simulink model "dspaudiosrc_fixpt"  (Simulink 8.3)
settings: Solver=FixedStepDiscrete  SolverMode=SingleTasking  StartTime=0.0  StopTime=inf  RelTol=1e-3
model workspace (MATLAB code in the model file):
  | load dspaudiosrc
libraries: dspmlti4 x1, dspsigops x1, dspsrcs4 x1, dspmisc x1
settings Model: Creator=The MathWorks Inc.  ExtModeAutoUpdateStatusClock=off
settings DataIOCC: SaveOutput=off  SignalLogging=off  SaveTime=off
settings OptimizationCC: InlineParams=on  ExpressionDepthLimit=2147483647  InitFltsAndDblsToZero=on
settings DebuggingCC: SignalResolutionControl=TryResolveAllWithWarning  SolverPrmCheckMsg=none  MultiTaskDSMMsg=warning  MultiTaskCondExecSysMsg=none  IntegerOverflowMsg=none  ParameterPrecisionLossMsg=none  FcnCallInpInsideContextMsg=UseLocalSettings
settings HardwareCC: ProdHWDeviceType=ASIC/FPGA  TargetHWDeviceType=32-bit Generic  ProdEqTarget=off
settings RTWCC: IncludeERTFirstTime=on

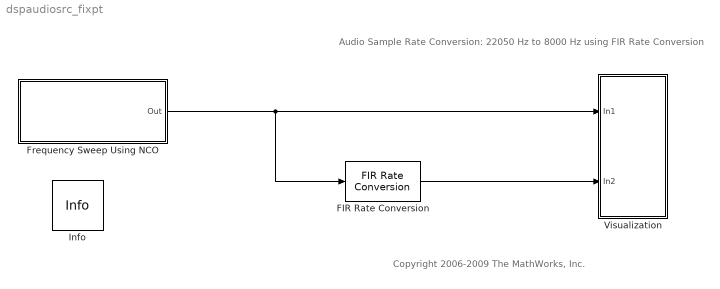
== system dspaudiosrc_fixpt ==
  note: Audio Sample Rate Conversion:
      | 22050 Hz to 8000 Hz using FIR Rate Conversion
  note: Copyright 2006-2009 The MathWorks, Inc.
  FIR Rate Conversion : dspmlti4/FIR Rate Conversion  Tag=BlockMethodSubSystem  L=160  h=b  M=441  firstCoeffMode=Specify word length  firstCoeffWordLength=16  firstCoeffFracLength=0  firstCoeffDataTypeStr=fixdt(1,16)  firstCoeffLastDataTypeStr=fixdt(1,16)  firstCoeffMin=[]  firstCoeffMax=[]  outputMode=Binary point scaling  outputWordLength=16  outputFracLength=15  outputDataTypeStr=fixdt(1,16,15)  outputLastDataTypeStr=fixdt(1,16,15)  outputMin=[]  outputMax=[]  accumMode=Binary point scaling  accumWordLength=32  accumFracLength=30  accumDataTypeStr=fixdt(1,32,30)  accumLastDataTypeStr=fixdt(1,32,30)  roundingMode=Nearest  overflowMode=on  FilterSource=Specify via dialog  FilterObject=Hm_firsrc
  Frequency Sweep Using NCO : Subsystem
      mask init:
      | t = [0:0.1:1.5*pi];
      | y = (sin(t.*t)+1)/2*0.7;
      | t = t / max(t);
      mask Display:
      | plot(t,y);
      | text(.2,.85,'Linear (0 - 22050 Hz)')
  Info : dspmisc/Info  SystemSampleTime=-1
  Visualization : Subsystem
      mask Display: disp('SCOPES')
  wires:
  FIR Rate Conversion/1 -> Visualization/2(In2)
  Frequency Sweep Using NCO/1(Out) -> Visualization/1(In1), FIR Rate Conversion/1

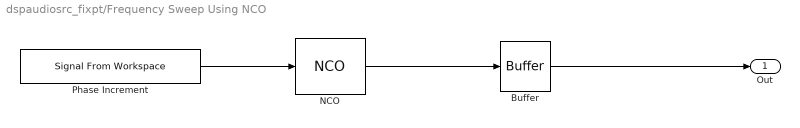
== system dspaudiosrc_fixpt/Frequency Sweep Using NCO ==
  Buffer : Buffer  N=441  TreatMby1Signals=One channel
  NCO : dspsigops/NCO  AccIncSrc=Input port  AccInc=1  PhaseOffsetSrc=Specify via dialog  PhaseOffset=0  AccumWL=32  HasDither=on  DitherWL=4  PNgeneratorLength=12  HasPhaseQuantizer=on  TableDepth=16  HasOutputPhaseError=off  Formula=Sine  DataType=Binary point scaling  OutputWL=16  OutputFL=15  CompMethod=Table lookup (no interpolation)  SampleTime=1/48000  SamplesPerFrame=1
  Phase Increment : dspsrcs4/Signal From Workspace  X=uint32((2^32)*(10000/22050) * (1/(10*22050):1/(10*22050):1))  Ts=1/22050  nsamps=1  OutputAfterFinalValue=Cyclic repetition  ignoreOrWarnInputAndFrameLengths=on
  Out : Outport
  wires:
  NCO/1 -> Buffer/1
  Phase Increment/1 -> NCO/1
  Buffer/1 -> Out/1

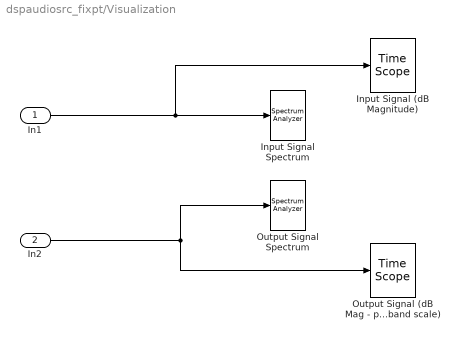
== system dspaudiosrc_fixpt/Visualization ==
  In1 : Inport
  In2 : Inport  Port=2
  Input Signal (dB Magnitude) : TimeScope  DefaultConfigurationName=spbscopes.TimeScopeBlockCfg  ScopeSpecification=DataTag0
  Input Signal Spectrum : SpectrumAnalyzer  ScopeSpecification=DataTag1
  Output Signal (dB Mag - passband scale) : TimeScope  DefaultConfigurationName=spbscopes.TimeScopeBlockCfg  ScopeSpecification=DataTag2
  Output Signal Spectrum : SpectrumAnalyzer  ScopeSpecification=DataTag3
  wires:
  In1/1 -> Input Signal Spectrum/1, Input Signal (dB Magnitude)/1
  In2/1 -> Output Signal Spectrum/1, Output Signal (dB Mag - passband scale)/1
